simulink library "ddm"  (R2021b)
settings: Solver=VariableStepAuto  StartTime=0.0  StopTime=10.0  RelTol=1e-3
undefined symbols (not defined in the file): ADDM_FrTMTqDev_X_Nm, ADDM_RrTMTqDev_X_Nm, ENUM_ADASACCSTA_ERROR, ENUM_ADASACCSTA_OFF, ENUM_ADASACCSTA_STANDBY, ENUM_ALLOWMOV_ALLOWREADY, ENUM_APS, ENUM_BRKSTA_ERROR, ENUM_BRKSTA_OFF, ENUM_BRKSTA_ON, ENUM_BRKSW_INVALID, ENUM_BRKSW_OFF, ENUM_BRKSW_ON, ENUM_CHGPREACTERRSTA_OBCPRE, ENUM_DCDCFAULTSTA_ANYFAULTLV1, ENUM_DCDCFAULTSTA_ANYFAULTLV2, ENUM_DRIVETRAIN_AWD, ENUM_DRIVETRAIN_FWD, ENUM_DRIVETRAIN_RWD, ENUM_EDUDRTSTA_NORMAL, ENUM_EPBERROR_FAILED, ENUM_EPBSTA_APPLIED, ENUM_EPBSTA_RELEASED, ENUM_ESCAPSSta_APSUNAVAILABLE, ENUM_GEARACTUALPOSN_INVALID, ENUM_GEARACTUALPOSN_P, ENUM_HVBATTREADYPRE_READY, ENUM_HWRESETSTA_HWRESETING, ENUM_MCUWARN_LV0, ENUM_MCUWARN_LV1, ENUM_MCUWARN_LV2, ENUM_MCUWARN_LV3, ENUM_MCUWARN_NOERROR, ENUM_OBCFAULTSTA_ANYFAULT, ENUM_PAS_R2F2, ENUM_PDFAULT_BATTPDFAIL, ENUM_PDFAULT_DCDCDISABLE, ENUM_PDFAULT_MCUDISABLE, ENUM_PDFAULT_MCUDISCHRG, ENUM_POWERSTA_OFF, ENUM_POWERSTA_ON, ENUM_POWERSTA_READY, ENUM_POWERSTA_STANDBY, ENUM_PRESSINDI_LOW, ENUM_PUFAULT_BATTUPFAIL, ENUM_PUFAULT_DCDCENABLEFAIL, ENUM_PUFAULT_PRECHRGCHKFAIL, ENUM_PUFAULT_SAFETYCHKFAIL, ENUM_PWRSTASW_OFF, ENUM_PWRSTASW_OFFA, ENUM_PWRSTASW_OFFCHVCHRG, ENUM_PWRSTASW_OFFCLVCHRG, ENUM_PWRSTASW_ON, ENUM_PWRSTASW_ONHVCHRG, ENUM_PWRSTASW_READY, ENUM_PWRSTASW_STANDBY, ENUM_RAPSErrWarnSta_NORMAL, ENUM_RAPSErrWarnSta_RAPSERRLV1, ENUM_SHIFTCOMMAND_P, ENUM_SHIFTERERRSTA_PBUTTONFAILURE ... (+471)
libraries: hcu_lib x540, simulink x3
(part 10 of 26)

== system ddm/DDM/DDM/PMM/power up and power down ==
  note: VDDM_EDriveSysErrPowerUp_flg
  note: Power up fail check
  note: Power down fail check
  note: OBC ready for precharge fail check
  note: VDDM_EDriveSysErrPowerUp_flg
  note: VDDM_EDriveSysErrPowerUp_flg
  note: VDDM_EDriveSysErrPowerUp_flg
  task_time_s : Inport
  VPMM_PwrStaSW_enum : Inport  Port=2
  VPMM_PowerSta_enum : Inport  Port=3
  VPMM_PowerUpFault_enum : Inport  Port=4
  VPMM_PowerDownFault_enum : Inport  Port=5
  DTC_clear_request : Inport  Port=6
  VINP_HVBattReady4Pre_enum : Inport  Port=7
  VDDM_RrMCUReady4Pre_flg : Inport  Port=8
  VINP_DCDCReady4Pre_flg : Inport  Port=9
  VINP_HVBContactorSta_flg : Inport  Port=10
  VINP_BMSREADY_flg : Inport  Port=11
  VINP_DCDCEnabled_flg : Inport  Port=12
  VPMM_SafetyChkHLv_flg : Inport  Port=13
  VPMM_SafetyChkMLv_flg : Inport  Port=14
  VPMM_HVChrgPreActionErrSta_enum : Inport  Port=15
  VDDM_RrMCUDCBusVolt_V : Inport  Port=16
  VDDM_ClearZevDTCcmd_flg : Inport  Port=17
  VDDM_FrMCUReady4Pre_flg : Inport  Port=18
  VDDM_RrMCUEnaSta_flg : Inport  Port=19
  VDDM_FrMCUEnaSta_flg : Inport  Port=20
  VDDM_FrMCUDCBusVolt_V : Inport  Port=21
  BMS HV relay closed fail : Subsystem
  BMS HV relay opened fail : Subsystem
  BMS ready fail : Subsystem
  DCDC disable fail : Subsystem
  DCDC enable fail : Subsystem
  DCDC ready for precharge fail : Subsystem
  Fr_MCU active discharge fail : Subsystem
  Fr_MCU disable fail : Subsystem
  Fr_MCU ready for precharge fail : Subsystem
  Ground : Ground
  HVB ready for precharge fail : Subsystem
  High level system safety check fail : Subsystem
  Logical Operator : Logic  Operator=OR  AllPortsSameDT=off  OutDataTypeStr=boolean
  Logical Operator1 : Logic  Operator=OR  Inputs=9  AllPortsSameDT=off  OutDataTypeStr=boolean
      settings: AttributesFormatString=%<Operator>
  Logical Operator2 : Logic  Operator=OR  Inputs=3  AllPortsSameDT=off  OutDataTypeStr=boolean
      settings: AttributesFormatString=%<Operator>
  Mid level system safety check fail : Subsystem
  OBC ready for precharge fail : Subsystem
  Rr_MCU active discharge fail : Subsystem
  Rr_MCU disable fail : Subsystem
  Rr_MCU ready for precharge fail : Subsystem
  VDDM_HVB4PreDTC_raw32 : Outport
  VDDM_MCU4PreDTC_raw32 : Outport  Port=2
  VDDM_DCDC4PreDTC_raw32 : Outport  Port=3
  VDDM_HVRlyCloDTC_raw32 : Outport  Port=4
  VDDM_BMSRdyDTC_raw32 : Outport  Port=5
  VDDM_DCDCEnaDTC_raw32 : Outport  Port=6
  VDDM_HiLvSaChkDTC_raw32 : Outport  Port=7
  VDDM_MidLvSaChkDTC_raw32 : Outport  Port=8
  VDDM_MCUDisDTC_raw32 : Outport  Port=9
  VDDM_DCDCDisDTC_raw32 : Outport  Port=10
  VDDM_HVRlyOpDTC_raw32 : Outport  Port=11
  VDDM_MCUActDTC_raw32 : Outport  Port=12
  VDDM_OBC4PreDTC_raw32 : Outport  Port=13
  VDDM_HVRlyOpFail_flg : Outport  Port=14
  VDDM_MCUActDisFail_flg : Outport  Port=15
  VDDM_HVB4PreCFS_flg : Outport  Port=16
  VDDM_RrMCU4PreCFS_flg : Outport  Port=17
  VDDM_DCDC4PreCFS_flg : Outport  Port=18
  VDDM_HVRlyCloCFS_flg : Outport  Port=19
  VDDM_BMSRdyCFS_flg : Outport  Port=20
  VDDM_DCDCEnaCFS_flg : Outport  Port=21
  VDDM_HiLvSaChkCFS_flg : Outport  Port=22
  VDDM_MidLvSaChkCFS_flg : Outport  Port=23
  VDDM_RrMCUDisCFS_flg : Outport  Port=24
  VDDM_DCDCDisCFS_flg : Outport  Port=25
  VDDM_HVRlyOpCFS_flg : Outport  Port=26
  VDDM_RrMCUActCFS_flg : Outport  Port=27
  VDDM_OBC4PreCFS_flg : Outport  Port=28
  VDDM_FrMCU4PreDTC_raw32 : Outport  Port=29
  VDDM_FrMCUDisDTC_ra32 : Outport  Port=30
  VDDM_FrMCUActDTC_raw32 : Outport  Port=31
  VDDM_FrMCU4PreCFS_flg : Outport  Port=32
  VDDM_FrMCUDisCFS_flg : Outport  Port=33
  VDDM_FrMCUActCFS_flg : Outport  Port=34
  VDDM_EDriveSysErrPowerUp_flg : Outport  Port=35
  VDDM_EDriveSysErrPowerDown_flg : Outport  Port=36
  VDDM_SystemPowerUpErr_flg : Outport  Port=37
  VDDM_SystemPowerDownErr_flg : Outport  Port=38
  wires:
  BMS HV relay closed fail/1(VDDM_HVRlyCloDTC_raw32) -> VDDM_HVRlyCloDTC_raw32/1
  DCDC ready for precharge fail/1(VDDM_DCDC4PreDTC_raw32) -> VDDM_DCDC4PreDTC_raw32/1
  Rr_MCU ready for precharge fail/1(VDDM_MCU4PreDTC_raw32) -> VDDM_MCU4PreDTC_raw32/1
  HVB ready for precharge fail/1(VDDM_HVB4PreDTC_raw32) -> VDDM_HVB4PreDTC_raw32/1
  BMS HV relay opened fail/2(VDDM_HVRlyOpFail_flg) -> VDDM_HVRlyOpFail_flg/1
  [VINP_HVBContactorSta_flg] -> BMS HV relay closed fail/4(VINP_HVBContactorSta_flg)
  VINP_HVBContactorSta_flg/1 -> [VINP_HVBContactorSta_flg]
  [VPMM_PowerDownFault_enum] -> Rr_MCU active discharge fail/4(VPMM_PowerDownFault_enum)
  [VPMM_PowerDownFault_enum] -> BMS HV relay opened fail/4(VPMM_PowerDownFault_enum)
  [VPMM_PowerDownFault_enum] -> DCDC disable fail/4(VPMM_PowerDownFault_enum)
  [VINP_DCDCEnabled_flg] -> DCDC enable fail/4(VINP_DCDCEnabled_flg)
  VINP_DCDCEnabled_flg/1 -> [VINP_DCDCEnabled_flg]
  [VPMM_PowerDownFault_enum] -> Rr_MCU disable fail/4(VPMM_PowerDownFault_enum)
  VPMM_PowerDownFault_enum/1 -> [VPMM_PowerDownFault_enum]
  [VPMM_PowerUpFault_enum] -> Mid level system safety check fail/5(VPMM_PowerUpFault_enum)
  VPMM_SafetyChkMLv_flg/1 -> Mid level system safety check fail/4(VDDM_MidLvSaChkChk_flg)
  High level system safety check fail/1(VDDM_HiLvSaChkDTC_raw32) -> VDDM_HiLvSaChkDTC_raw32/1
  VPMM_SafetyChkHLv_flg/1 -> High level system safety check fail/4(VPMM_SafetyChkHLv_flg)
  [VPMM_PowerSta_enum] -> High level system safety check fail/3(VPMM_PwrStaSW_enum)
  [DTC_clear_request] -> High level system safety check fail/6(DTC_clear_request)
  [VPMM_PowerUpFault_enum] -> High level system safety check fail/5(VPMM_PowerUpFault_enum)
  [VPMM_PwrStaSW_enum] -> High level system safety check fail/2(VPMM_PowerSta_enum)
  [task_time_s] -> High level system safety check fail/1(task_time_s)
  DCDC enable fail/1(VDDM_DCDCEnaDTC_raw32) -> VDDM_DCDCEnaDTC_raw32/1
  [VPMM_PowerSta_enum] -> DCDC enable fail/3(VPMM_PwrStaSW_enum)
  [VPMM_PwrStaSW_enum] -> DCDC enable fail/2(VPMM_PowerSta_enum)
  [VDDM_ClearZevDTCcmd_flg] -> DCDC enable fail/6(DTC_clear_request)
  [VPMM_PowerUpFault_enum] -> DCDC enable fail/5(VPMM_PowerUpFault_enum)
  [task_time_s] -> DCDC enable fail/1(task_time_s)
  BMS ready fail/1(VDDM_BMSRdyDTC_raw32) -> VDDM_BMSRdyDTC_raw32/1
  VINP_BMSREADY_flg/1 -> BMS ready fail/4(VINP_BMSREADY_flg)
  [VPMM_PowerSta_enum] -> BMS ready fail/3(VPMM_PwrStaSW_enum)
  [VPMM_PwrStaSW_enum] -> BMS ready fail/2(VPMM_PowerSta_enum)
  [VDDM_ClearZevDTCcmd_flg] -> BMS ready fail/6(DTC_clear_request)
  [VPMM_PowerUpFault_enum] -> BMS ready fail/5(VPMM_PowerUpFault_enum)
  [task_time_s] -> BMS ready fail/1(task_time_s)
  [VPMM_PowerUpFault_enum] -> BMS HV relay closed fail/5(VPMM_PowerUpFault_enum)
  [VPMM_PowerUpFault_enum] -> DCDC ready for precharge fail/5(VPMM_PowerUpFault_enum)
  [VPMM_PowerUpFault_enum] -> Rr_MCU ready for precharge fail/4(VPMM_PowerUpFault_enum)
  [VDDM_ClearZevDTCcmd_flg] -> Rr_MCU ready for precharge fail/5(DTC_clear_request)
  [VPMM_PowerUpFault_enum] -> HVB ready for precharge fail/5(VPMM_PowerUpFault_enum)
  VPMM_HVChrgPreActionErrSta_enum/1 -> OBC ready for precharge fail/4(VPMM_HVChrgPreActionErrSta_enum)
  VINP_DCDCReady4Pre_flg/1 -> DCDC ready for precharge fail/4(VINP_DCDCReady4Pre_flg)
  VINP_HVBattReady4Pre_enum/1 -> HVB ready for precharge fail/4(VINP_HVBattReady4Pre_enum)
  Rr_MCU active discharge fail/1(VDDM_MCUActDTC_raw32) -> VDDM_MCUActDTC_raw32/1
  Rr_MCU disable fail/1(VDDM_MCUDisDTC_raw32) -> VDDM_MCUDisDTC_raw32/1
  Mid level system safety check fail/1(VDDM_MidLvSaChkDTC_raw32) -> VDDM_MidLvSaChkDTC_raw32/1
  BMS HV relay opened fail/1(VDDM_HVRlyOpDTC_raw32) -> VDDM_HVRlyOpDTC_raw32/1
  OBC ready for precharge fail/1(VDDM_OBC4PreDTC_raw32) -> VDDM_OBC4PreDTC_raw32/1
  DCDC disable fail/1(VDDM_DCDCDisDTC_raw32) -> VDDM_DCDCDisDTC_raw32/1
  [VDDM_ClearZevDTCcmd_flg] -> OBC ready for precharge fail/5(DTC_clear_request)
  [task_time_s] -> OBC ready for precharge fail/1(task_time_s)
  [task_time_s] -> Rr_MCU active discharge fail/1(task_time_s)
  [VPMM_PwrStaSW_enum] -> Rr_MCU active discharge fail/3(VPMM_PwrStaSW_enum)
  [VDDM_ClearZevDTCcmd_flg] -> Rr_MCU active discharge fail/5(DTC_clear_request)
  [VPMM_PowerSta_enum] -> Rr_MCU active discharge fail/2(VPMM_PowerSta_enum)
  [VPMM_PowerSta_enum] -> BMS HV relay opened fail/2(VPMM_PowerSta_enum)
  [VDDM_ClearZevDTCcmd_flg] -> BMS HV relay opened fail/5(DTC_clear_request)
  [VPMM_PwrStaSW_enum] -> BMS HV relay opened fail/3(VPMM_PwrStaSW_enum)
  [task_time_s] -> BMS HV relay opened fail/1(task_time_s)
  [task_time_s] -> DCDC disable fail/1(task_time_s)
  [VDDM_ClearZevDTCcmd_flg] -> DCDC disable fail/5(DTC_clear_request)
  [VPMM_PowerSta_enum] -> Rr_MCU disable fail/2(VPMM_PowerSta_enum)
  [VDDM_ClearZevDTCcmd_flg] -> Rr_MCU disable fail/5(DTC_clear_request)
  [VPMM_PwrStaSW_enum] -> Rr_MCU disable fail/3(VPMM_PwrStaSW_enum)
  [task_time_s] -> Rr_MCU disable fail/1(task_time_s)
  [task_time_s] -> Mid level system safety check fail/1(task_time_s)
  [VPMM_PwrStaSW_enum] -> Mid level system safety check fail/2(VPMM_PowerSta_enum)
  [DTC_clear_request] -> Mid level system safety check fail/6(DTC_clear_request)
  [VPMM_PowerSta_enum] -> Mid level system safety check fail/3(VPMM_PwrStaSW_enum)
  DTC_clear_request/1 -> [DTC_clear_request]
  VPMM_PowerSta_enum/1 -> [VPMM_PowerSta_enum]
  task_time_s/1 -> [task_time_s]
  VPMM_PwrStaSW_enum/1 -> [VPMM_PwrStaSW_enum]
  VPMM_PowerUpFault_enum/1 -> [VPMM_PowerUpFault_enum]
  [task_time_s] -> Rr_MCU ready for precharge fail/1(task_time_s)
  [VPMM_PwrStaSW_enum] -> HVB ready for precharge fail/2(VPMM_PowerSta_enum)
  [VPMM_PwrStaSW_enum] -> BMS HV relay closed fail/2(VPMM_PowerSta_enum)
  [VPMM_PowerSta_enum] -> BMS HV relay closed fail/3(VPMM_PwrStaSW_enum)
  [task_time_s] -> BMS HV relay closed fail/1(task_time_s)
  [VPMM_PowerSta_enum] -> Rr_MCU ready for precharge fail/3(VPMM_PwrStaSW_enum)
  [VPMM_PwrStaSW_enum] -> DCDC ready for precharge fail/2(VPMM_PowerSta_enum)
  [task_time_s] -> DCDC ready for precharge fail/1(task_time_s)
  [VDDM_ClearZevDTCcmd_flg] -> DCDC ready for precharge fail/6(VINP_ReqClrDTC_flg)
  [task_time_s] -> HVB ready for precharge fail/1(task_time_s)
  [VDDM_ClearZevDTCcmd_flg] -> HVB ready for precharge fail/6(DTC_clear_request)
  [VPMM_PowerSta_enum] -> HVB ready for precharge fail/3(VPMM_PwrStaSW_enum)
  [VPMM_PowerSta_enum] -> DCDC ready for precharge fail/3(VPMM_PwrStaSW_enum)
  [VPMM_PwrStaSW_enum] -> Rr_MCU ready for precharge fail/2(VPMM_PowerSta_enum)
  [VDDM_ClearZevDTCcmd_flg] -> BMS HV relay closed fail/6(DTC_clear_request)
  [VDDM_RrMCUDCBusVolt_V] -> Rr_MCU active discharge fail/6(VDDM_RrMCUDCBusVolt_V)
  HVB ready for precharge fail/2(VDDM_HVB4PreCFS_flg) -> [VDDM_HVB4PreCFS_flg]
  Rr_MCU ready for precharge fail/2(VDDM_RrMCU4PreCFS_flg) -> [VDDM_RrMCU4PreCFS_flg]
  DCDC ready for precharge fail/2(VDDM_DCDC4PreCFS_flg) -> [VDDM_DCDC4PreCFS_flg]
  BMS HV relay closed fail/2(VDDM_HVRlyCloCFS_flg) -> [VDDM_HVRlyCloCFS_flg]
  BMS ready fail/2(VDDM_BMSRdyCFS_flg) -> [VDDM_BMSRdyCFS_flg]
  DCDC enable fail/2(VDDM_DCDCEnaCFS_flg) -> [VDDM_DCDCEnaCFS_flg]
  High level system safety check fail/2(VDDM_HiLvSaChkCFS_flg) -> [VDDM_HiLvSaChkCFS_flg]
  Mid level system safety check fail/2(VDDM_MidLvSaChkCFS_flg) -> [VDDM_MidLvSaChkCFS_flg]
  Rr_MCU disable fail/2(VDDM_RrMCUDisCFS_flg) -> [VDDM_RrMCUDisCFS_flg]
  DCDC disable fail/2(VDDM_DCDCDisCFS_flg) -> [VDDM_DCDCDisCFS_flg]
  BMS HV relay opened fail/3(VDDM_HVRlyOpCFS_flg) -> [VDDM_HVRlyOpCFS_flg]
  Rr_MCU active discharge fail/3(VDDM_RrMCUActCFS_flg) -> [VDDM_RrMCUActCFS_flg]
  OBC ready for precharge fail/2(VDDM_OBC4PreCFS_flg) -> [VDDM_OBC4PreCFS_flg]
  [VDDM_HVB4PreCFS_flg] -> VDDM_HVB4PreCFS_flg/1
  [VDDM_RrMCU4PreCFS_flg] -> VDDM_RrMCU4PreCFS_flg/1
  [VDDM_DCDC4PreCFS_flg] -> VDDM_DCDC4PreCFS_flg/1
  [VDDM_HVRlyCloCFS_flg] -> VDDM_HVRlyCloCFS_flg/1
  [VDDM_BMSRdyCFS_flg] -> VDDM_BMSRdyCFS_flg/1
  [VDDM_DCDCEnaCFS_flg] -> VDDM_DCDCEnaCFS_flg/1
  [VDDM_HiLvSaChkCFS_flg] -> VDDM_HiLvSaChkCFS_flg/1
  [VDDM_MidLvSaChkCFS_flg] -> VDDM_MidLvSaChkCFS_flg/1
  [VDDM_RrMCUDisCFS_flg] -> VDDM_RrMCUDisCFS_flg/1
  [VDDM_DCDCDisCFS_flg] -> VDDM_DCDCDisCFS_flg/1
  [VDDM_HVRlyOpCFS_flg] -> VDDM_HVRlyOpCFS_flg/1
  [VDDM_RrMCUActCFS_flg] -> VDDM_RrMCUActCFS_flg/1
  [VDDM_OBC4PreCFS_flg] -> VDDM_OBC4PreCFS_flg/1
  VDDM_RrMCUDCBusVolt_V/1 -> [VDDM_RrMCUDCBusVolt_V]
  VDDM_ClearZevDTCcmd_flg/1 -> [VDDM_ClearZevDTCcmd_flg]
  [VDDM_FrMCUReady4Pre_flg] -> Fr_MCU ready for precharge fail/6(VDDM_FrMCUReady4Pre_flg)
  [DTC_clear_request] -> Fr_MCU ready for precharge fail/5(DTC_clear_request)
  [VPMM_PowerSta_enum] -> Fr_MCU ready for precharge fail/3(VPMM_PwrStaSW_enum)
  [task_time_s] -> Fr_MCU ready for precharge fail/1(task_time_s)
  Fr_MCU ready for precharge fail/2(VDDM_FrMCU4PreCFS_flg) -> [VDDM_FrMCU4PreCFS_flg]
  [VPMM_PowerUpFault_enum] -> Fr_MCU ready for precharge fail/4(VPMM_PowerUpFault_enum)
  [VPMM_PwrStaSW_enum] -> Fr_MCU ready for precharge fail/2(VPMM_PowerSta_enum)
  Fr_MCU ready for precharge fail/1(VDDM_FrMCU4PreDTC_raw32) -> VDDM_FrMCU4PreDTC_raw32/1
  Ground/1 -> [VPMM_PowerUpState_enum]
  [VDDM_RrMCUEnaSta_flg] -> Rr_MCU disable fail/6(VDDM_RrMCUEnaSta_flg)
  [VPMM_PowerSta_enum] -> DCDC disable fail/2(VPMM_PowerSta_enum)
  [VPMM_PwrStaSW_enum] -> DCDC disable fail/3(VPMM_PwrStaSW_enum)
  Rr_MCU active discharge fail/2(VDDM_RrMCUActDisFail_flg) -> [VDDM_RrMCUActDisFail_flg]
  [VPMM_PowerSta_enum] -> Fr_MCU disable fail/3(VPMM_PwrStaSW_enum)
  [task_time_s] -> Fr_MCU disable fail/1(task_time_s)
  [VDDM_FrMCUEnaSta_flg] -> Fr_MCU disable fail/6(VDDM_FrMCUEnaSta_flg)
  Fr_MCU disable fail/1(VDDM_FrMCUDisDTC_raw32) -> VDDM_FrMCUDisDTC_ra32/1
  [DTC_clear_request] -> Fr_MCU disable fail/5(DTC_clear_request)
  Fr_MCU disable fail/2(VDDM_FrMCUDisCFS_flg) -> [VDDM_FrMCUDisCFS_flg]
  [VPMM_PowerDownFault_enum] -> Fr_MCU disable fail/4(VPMM_PowerDownFault_enum)
  [VPMM_PwrStaSW_enum] -> Fr_MCU disable fail/2(VPMM_PowerSta_enum)
  [VPMM_PwrStaSW_enum] -> Fr_MCU active discharge fail/3(VPMM_PwrStaSW_enum)
  Fr_MCU active discharge fail/2(VDDM_FrMCUActDisFail_flg) -> [VDDM_FrMCUActDisFail_flg]
  [VPMM_PowerSta_enum] -> Fr_MCU active discharge fail/2(VPMM_PowerSta_enum)
  [task_time_s] -> Fr_MCU active discharge fail/1(task_time_s)
  [DTC_clear_request] -> Fr_MCU active discharge fail/5(DTC_clear_request)
  Fr_MCU active discharge fail/3(VDDM_FrMCUActCFS_flg) -> [VDDM_FrMCUActCFS_flg]
  Fr_MCU active discharge fail/1(VDDM_FrMCUActDTC_raw32) -> VDDM_FrMCUActDTC_raw32/1
  [VDDM_FrMCUDCBusVolt_V] -> Fr_MCU active discharge fail/6(VDDM_FrMCUDCBusVolt_V)
  [VPMM_PowerDownFault_enum] -> Fr_MCU active discharge fail/4(VPMM_PowerDownFault_enum)
  [VDDM_RrMCUActDisFail_flg] -> Logical Operator/2
  [VDDM_FrMCUActDisFail_flg] -> Logical Operator/1
  Logical Operator/1 -> VDDM_MCUActDisFail_flg/1  "VDDM_MCUActDisFail_flg"
  [VPMM_PowerSta_enum] -> OBC ready for precharge fail/2(VPMM_PowerSta_enum)
  [VPMM_PwrStaSW_enum] -> OBC ready for precharge fail/3(VPMM_PwrStaSW_enum)
  [VDDM_FrMCUDisCFS_flg] -> VDDM_FrMCUDisCFS_flg/1
  [VDDM_FrMCU4PreCFS_flg] -> VDDM_FrMCU4PreCFS_flg/1
  [VDDM_FrMCUActCFS_flg] -> VDDM_FrMCUActCFS_flg/1
  Logical Operator2/1 -> [VDDM_EDriveSysErrPowerDown_flg], [VDDM_SystemPowerDownErr_flg]  "VDDM_EDriveSysErrPowerDown_flg"
  [VDDM_FrMCU4PreCFS_flg] -> Logical Operator1/3
  [VDDM_FrMCUActCFS_flg] -> Logical Operator2/2
  [VDDM_HVRlyOpCFS_flg] -> Logical Operator2/1
  [VDDM_MidLvSaChkCFS_flg] -> Logical Operator1/9
  [VDDM_DCDC4PreCFS_flg] -> Logical Operator1/4
  [VDDM_HVRlyCloCFS_flg] -> Logical Operator1/5
  Logical Operator1/1 -> [VDDM_EDriveSysErrPowerUp_flg], [VDDM_SystemPowerUpErr_flg]  "VDDM_EDriveSysErrPowerUp_flg"
  [VDDM_HiLvSaChkCFS_flg] -> Logical Operator1/8
  [VDDM_HVB4PreCFS_flg] -> Logical Operator1/1
  [VDDM_BMSRdyCFS_flg] -> Logical Operator1/6
  [VDDM_DCDCEnaCFS_flg] -> Logical Operator1/7
  [VDDM_RrMCUActCFS_flg] -> Logical Operator2/3
  [VDDM_RrMCU4PreCFS_flg] -> Logical Operator1/2
  [VDDM_EDriveSysErrPowerUp_flg] -> VDDM_EDriveSysErrPowerUp_flg/1
  [VDDM_EDriveSysErrPowerDown_flg] -> VDDM_EDriveSysErrPowerDown_flg/1
  [VDDM_RrMCUReady4Pre_flg] -> Rr_MCU ready for precharge fail/6(VDDM_RrMCUReady4Pre_flg)
  VDDM_RrMCUReady4Pre_flg/1 -> [VDDM_RrMCUReady4Pre_flg]
  VDDM_FrMCUReady4Pre_flg/1 -> [VDDM_FrMCUReady4Pre_flg]
  VDDM_RrMCUEnaSta_flg/1 -> [VDDM_RrMCUEnaSta_flg]
  VDDM_FrMCUEnaSta_flg/1 -> [VDDM_FrMCUEnaSta_flg]
  VDDM_FrMCUDCBusVolt_V/1 -> [VDDM_FrMCUDCBusVolt_V]
  [VDDM_SystemPowerDownErr_flg] -> VDDM_SystemPowerDownErr_flg/1
  [VDDM_SystemPowerUpErr_flg] -> VDDM_SystemPowerUpErr_flg/1

== system ddm/DDM/DDM/Subsystem/Subsystem ==
  VPMM_SysPwrSta_enum : Inport
  VINP_CANBusError_flg : Inport  Port=2
  Constant17 : Constant  Value=ENUM_PWRSTASW_READY
  Constant3 : Constant  Value=ENUM_PWRSTASW_ON
  Equal2 : RelationalOperator  Operator===  OutDataTypeStr=boolean  RndMeth=Simplest
  Equal6 : RelationalOperator  Operator===  OutDataTypeStr=boolean  RndMeth=Simplest
  Logical Operator1 : Logic  AllPortsSameDT=off  OutDataTypeStr=boolean
  Logical Operator13 : Logic  Operator=OR  AllPortsSameDT=off  OutDataTypeStr=boolean
  Logical Operator2 : Logic  AllPortsSameDT=off  OutDataTypeStr=boolean
  NOT : Logic  Operator=NOT  AllPortsSameDT=off  OutDataTypeStr=boolean
  VDDM_CANBusErrorPass_flg : Outport
  VDDM_CANBusErrorCFS_flg : Outport  Port=2
  wires:
  Equal6/1 -> Logical Operator13/1
  [VPMM_SysPwrSta_enum] -> Equal6/1
  Equal2/1 -> Logical Operator13/2
  [VPMM_SysPwrSta_enum] -> Equal2/1
  Constant3/1 -> Equal6/2
  Constant17/1 -> Equal2/2
  VPMM_SysPwrSta_enum/1 -> [VPMM_SysPwrSta_enum]
  VINP_CANBusError_flg/1 -> [VINP_CANBusError_flg]
  Logical Operator13/1 -> Logical Operator2/1, Logical Operator1/1
  [VINP_CANBusError_flg] -> NOT/1, Logical Operator1/2
  Logical Operator1/1 -> VDDM_CANBusErrorCFS_flg/1
  NOT/1 -> Logical Operator2/2
  Logical Operator2/1 -> VDDM_CANBusErrorPass_flg/1

== system ddm/DDM/DDM/Subsystem/Subsystem1 ==
  VPMM_SysPwrSta_enum : Inport
  VINP_CANBusError_flg : Inport  Port=2
  Constant17 : Constant  Value=ENUM_PWRSTASW_READY
  Constant3 : Constant  Value=ENUM_PWRSTASW_ON
  Equal2 : RelationalOperator  Operator===  OutDataTypeStr=boolean  RndMeth=Simplest
  Equal6 : RelationalOperator  Operator===  OutDataTypeStr=boolean  RndMeth=Simplest
  Logical Operator1 : Logic  AllPortsSameDT=off  OutDataTypeStr=boolean
  Logical Operator13 : Logic  Operator=OR  AllPortsSameDT=off  OutDataTypeStr=boolean
  Logical Operator2 : Logic  AllPortsSameDT=off  OutDataTypeStr=boolean
  NOT : Logic  Operator=NOT  AllPortsSameDT=off  OutDataTypeStr=boolean
  VDDM_CANBusErrorPass_flg : Outport
  VDDM_CANBusErrorCFS_flg : Outport  Port=2
  wires:
  Logical Operator2/1 -> VDDM_CANBusErrorPass_flg/1
  NOT/1 -> Logical Operator2/2
  Logical Operator1/1 -> VDDM_CANBusErrorCFS_flg/1
  [VINP_CANBusError_flg] -> Logical Operator1/2, NOT/1
  Logical Operator13/1 -> Logical Operator1/1, Logical Operator2/1
  VINP_CANBusError_flg/1 -> [VINP_CANBusError_flg]
  VPMM_SysPwrSta_enum/1 -> [VPMM_SysPwrSta_enum]
  Constant17/1 -> Equal2/2
  Constant3/1 -> Equal6/2
  [VPMM_SysPwrSta_enum] -> Equal2/1
  Equal2/1 -> Logical Operator13/2
  [VPMM_SysPwrSta_enum] -> Equal6/1
  Equal6/1 -> Logical Operator13/1

== system ddm/DDM/DDM/Subsystem/Subsystem2 ==
  VPMM_SysPwrSta_enum : Inport
  VINP_CANBusError_flg : Inport  Port=2
  Constant17 : Constant  Value=ENUM_PWRSTASW_READY
  Constant3 : Constant  Value=ENUM_PWRSTASW_ON
  Equal2 : RelationalOperator  Operator===  OutDataTypeStr=boolean  RndMeth=Simplest
  Equal6 : RelationalOperator  Operator===  OutDataTypeStr=boolean  RndMeth=Simplest
  Logical Operator1 : Logic  AllPortsSameDT=off  OutDataTypeStr=boolean
  Logical Operator13 : Logic  Operator=OR  AllPortsSameDT=off  OutDataTypeStr=boolean
  Logical Operator2 : Logic  AllPortsSameDT=off  OutDataTypeStr=boolean
  NOT : Logic  Operator=NOT  AllPortsSameDT=off  OutDataTypeStr=boolean
  VDDM_CANBusErrorPass_flg : Outport
  VDDM_CANBusErrorCFS_flg : Outport  Port=2
  wires:
  Logical Operator2/1 -> VDDM_CANBusErrorPass_flg/1
  NOT/1 -> Logical Operator2/2
  Logical Operator1/1 -> VDDM_CANBusErrorCFS_flg/1
  [VINP_CANBusError_flg] -> Logical Operator1/2, NOT/1
  Logical Operator13/1 -> Logical Operator1/1, Logical Operator2/1
  VINP_CANBusError_flg/1 -> [VINP_CANBusError_flg]
  VPMM_SysPwrSta_enum/1 -> [VPMM_SysPwrSta_enum]
  Constant17/1 -> Equal2/2
  Constant3/1 -> Equal6/2
  [VPMM_SysPwrSta_enum] -> Equal2/1
  Equal2/1 -> Logical Operator13/2
  [VPMM_SysPwrSta_enum] -> Equal6/1
  Equal6/1 -> Logical Operator13/1

== system ddm/DDM/DDM/Subsystem/Subsystem3 ==
  VPMM_SysPwrSta_enum : Inport
  VINP_CANBusError_flg : Inport  Port=2
  Constant17 : Constant  Value=ENUM_PWRSTASW_READY
  Constant3 : Constant  Value=ENUM_PWRSTASW_ON
  Equal2 : RelationalOperator  Operator===  OutDataTypeStr=boolean  RndMeth=Simplest
  Equal6 : RelationalOperator  Operator===  OutDataTypeStr=boolean  RndMeth=Simplest
  Logical Operator1 : Logic  AllPortsSameDT=off  OutDataTypeStr=boolean
  Logical Operator13 : Logic  Operator=OR  AllPortsSameDT=off  OutDataTypeStr=boolean
  Logical Operator2 : Logic  AllPortsSameDT=off  OutDataTypeStr=boolean
  NOT : Logic  Operator=NOT  AllPortsSameDT=off  OutDataTypeStr=boolean
  VDDM_CANBusErrorPass_flg : Outport
  VDDM_CANBusErrorCFS_flg : Outport  Port=2
  wires:
  Logical Operator2/1 -> VDDM_CANBusErrorPass_flg/1
  NOT/1 -> Logical Operator2/2
  Logical Operator1/1 -> VDDM_CANBusErrorCFS_flg/1
  [VINP_CANBusError_flg] -> Logical Operator1/2, NOT/1
  Logical Operator13/1 -> Logical Operator1/1, Logical Operator2/1
  VINP_CANBusError_flg/1 -> [VINP_CANBusError_flg]
  VPMM_SysPwrSta_enum/1 -> [VPMM_SysPwrSta_enum]
  Constant17/1 -> Equal2/2
  Constant3/1 -> Equal6/2
  [VPMM_SysPwrSta_enum] -> Equal2/1
  Equal2/1 -> Logical Operator13/2
  [VPMM_SysPwrSta_enum] -> Equal6/1
  Equal6/1 -> Logical Operator13/1

== system ddm/DDM/DDM/Subsystem/Subsystem4 ==
  VPMM_SysPwrSta_enum : Inport
  VINP_CANBusError_flg : Inport  Port=2
  Constant17 : Constant  Value=ENUM_PWRSTASW_READY
  Constant3 : Constant  Value=ENUM_PWRSTASW_ON
  Equal2 : RelationalOperator  Operator===  OutDataTypeStr=boolean  RndMeth=Simplest
  Equal6 : RelationalOperator  Operator===  OutDataTypeStr=boolean  RndMeth=Simplest
  Logical Operator1 : Logic  AllPortsSameDT=off  OutDataTypeStr=boolean
  Logical Operator13 : Logic  Operator=OR  AllPortsSameDT=off  OutDataTypeStr=boolean
  Logical Operator2 : Logic  AllPortsSameDT=off  OutDataTypeStr=boolean
  NOT : Logic  Operator=NOT  AllPortsSameDT=off  OutDataTypeStr=boolean
  VDDM_CANBusErrorPass_flg : Outport
  VDDM_CANBusErrorCFS_flg : Outport  Port=2
  wires:
  Logical Operator2/1 -> VDDM_CANBusErrorPass_flg/1
  NOT/1 -> Logical Operator2/2
  Logical Operator1/1 -> VDDM_CANBusErrorCFS_flg/1
  [VINP_CANBusError_flg] -> Logical Operator1/2, NOT/1
  Logical Operator13/1 -> Logical Operator1/1, Logical Operator2/1
  VINP_CANBusError_flg/1 -> [VINP_CANBusError_flg]
  VPMM_SysPwrSta_enum/1 -> [VPMM_SysPwrSta_enum]
  Constant17/1 -> Equal2/2
  Constant3/1 -> Equal6/2
  [VPMM_SysPwrSta_enum] -> Equal2/1
  Equal2/1 -> Logical Operator13/2
  [VPMM_SysPwrSta_enum] -> Equal6/1
  Equal6/1 -> Logical Operator13/1

== system ddm/DDM/DDM/Subsystem/Subsystem5 ==
  VPMM_SysPwrSta_enum : Inport
  VINP_CANBusError_flg : Inport  Port=2
  Constant17 : Constant  Value=ENUM_PWRSTASW_READY
  Constant3 : Constant  Value=ENUM_PWRSTASW_ON
  Equal2 : RelationalOperator  Operator===  OutDataTypeStr=boolean  RndMeth=Simplest
  Equal6 : RelationalOperator  Operator===  OutDataTypeStr=boolean  RndMeth=Simplest
  Logical Operator1 : Logic  AllPortsSameDT=off  OutDataTypeStr=boolean
  Logical Operator13 : Logic  Operator=OR  AllPortsSameDT=off  OutDataTypeStr=boolean
  Logical Operator2 : Logic  AllPortsSameDT=off  OutDataTypeStr=boolean
  NOT : Logic  Operator=NOT  AllPortsSameDT=off  OutDataTypeStr=boolean
  VDDM_CANBusErrorPass_flg : Outport
  VDDM_CANBusErrorCFS_flg : Outport  Port=2
  wires:
  Logical Operator2/1 -> VDDM_CANBusErrorPass_flg/1
  NOT/1 -> Logical Operator2/2
  Logical Operator1/1 -> VDDM_CANBusErrorCFS_flg/1
  [VINP_CANBusError_flg] -> Logical Operator1/2, NOT/1
  Logical Operator13/1 -> Logical Operator1/1, Logical Operator2/1
  VINP_CANBusError_flg/1 -> [VINP_CANBusError_flg]
  VPMM_SysPwrSta_enum/1 -> [VPMM_SysPwrSta_enum]
  Constant17/1 -> Equal2/2
  Constant3/1 -> Equal6/2
  [VPMM_SysPwrSta_enum] -> Equal2/1
  Equal2/1 -> Logical Operator13/2
  [VPMM_SysPwrSta_enum] -> Equal6/1
  Equal6/1 -> Logical Operator13/1

== system ddm/DDM/DDM/TPM/LFBatwarn ==
  note: Test Detection Criteria
  note: Test Pass Criteria
  note: Release Condition After Decision
  note: Diagnostics and Fault Handling
  task_time_s : Inport
  VPMM_PowerSta_enum : Inport  Port=2
  DTC_clear_request : Inport  Port=3
  VTPM_LFBatwarn_flg : Inport  Port=4
  Constant : Constant  Value=KDDM_LFBatwarnDTC_cnt
  Constant1 : Constant  Value=KDDM_LFBatwarnDTC_cnt
  Constant10 : Constant  Value=ENUM_POWERSTA_OFF
  Constant11 : Constant  Value=KDDM_LFBatwarnPassSW_flg
  Constant12 : Constant  Value=FALSE
  Constant13 : Constant  Value=KDDM_LFBatwarnCFSSW_flg
  Constant14 : Constant  Value=KDDM_LFBatwarnDFSSW_flg
  Constant15 : Constant  Value=KDDM_LFBatwarnPassTO_s
  Constant2 : Constant  Value=ENUM_POWERSTA_READY
  Constant24 : Constant  Value=TRUE
  Constant25 : Constant  Value=FALSE
  Constant3 : Constant  Value=ENUM_POWERSTA_ON
  Constant4 : Constant  Value=FALSE
  Constant46 : Constant  Value=KDDM_LFBatwarnDetSW_flg
  Constant5 : Constant  Value=ENUM_POWERSTA_READY
  Constant6 : Constant  Value=KDDM_LFBatwarnDetTO_s
  Constant7 : Constant  Value=ENUM_POWERSTA_ON
  Constant8 : Constant  Value=TRUE
  Constant9 : Constant  Value=KDDM_LFBatwarnPassTO_s
  DTC_Couter : hcu_lib/Basic_Blocks/DTC_Couter
  DTC_Info : hcu_lib/Basic_Blocks/DTC_Info
  Data Type Conversion1 : DataTypeConversion  OutDataTypeStr=uint8
  Equal{1..5} (5 alike) : RelationalOperator  Operator===  OutDataTypeStr=boolean  RndMeth=Simplest
  Equal6 : RelationalOperator  OutDataTypeStr=boolean  RndMeth=Simplest
  Logical Operator{1,4..5,7..8} (5 alike) : Logic  Operator=OR  AllPortsSameDT=off  OutDataTypeStr=boolean
  Logical Operator12 : Logic  AllPortsSameDT=off  OutDataTypeStr=boolean
  Logical Operator15 : Logic  AllPortsSameDT=off  OutDataTypeStr=boolean
  Logical Operator18 : Logic  AllPortsSameDT=off  OutDataTypeStr=boolean
  Logical Operator19 : Logic  Inputs=3  AllPortsSameDT=off  OutDataTypeStr=boolean
  Logical Operator2 : Logic  Operator=NOT  AllPortsSameDT=off  OutDataTypeStr=boolean
  Logical Operator3 : Logic  Operator=OR  Inputs=3  AllPortsSameDT=off  OutDataTypeStr=boolean
  Logical Operator6 : Logic  Operator=NOT  AllPortsSameDT=off  OutDataTypeStr=boolean
  Relay : Relay  OnSwitchValue=ONE_INT  OffSwitchValue=ZERO_INT
  SR_Latch1 : Subsystem  mask(SR_Latch){}
      mask help: SR latch function.
  SR_Latch3 : hcu_lib/Basic_Blocks/SR_Latch
  SR_Latch4 : hcu_lib/Basic_Blocks/SR_Latch
  Switch{2..4,6} (4 alike) : Switch  Criteria=u2 ~= 0
  Test Detection Criteria : hcu_lib/Basic_Blocks/Test Detection Criteria
  Timer1 : hcu_lib/Basic_Blocks/Timer
  VDDM_LFBatwarnDTC_raw32 : Outport
  wires:
  task_time_s/1 -> [task_time_s]
  VPMM_PowerSta_enum/1 -> [VPMM_PowerSta_enum]
  Logical Operator8/1 -> Switch2/2
  Constant25/1 -> Switch2/3
  Switch2/1 -> [VDDM_LFBatwarnCFSRls_flg]
  [DTC_clear_request] -> Logical Operator8/2
  Constant24/1 -> Switch2/1
  Constant10/1 -> Equal4/2
  Equal4/1 -> Logical Operator8/1
  [VDDM_LFBatwarnDTC_cnt] -> Relay/1
  [VDDM_LFBatwarnCFS_flg] -> Logical Operator7/1
  Logical Operator3/1 -> Logical Operator15/1
  [VDDM_LFBatwarnDet_flg] -> Logical Operator19/1
  Relay/1 -> SR_Latch3/1
  DTC_Couter/2 -> Data Type Conversion1/1
  Logical Operator15/1 -> DTC_Couter/2
  Constant11/1 -> Logical Operator15/2
  Logical Operator19/1 -> DTC_Couter/1
  Constant46/1 -> Logical Operator19/2
  Data Type Conversion1/1 -> [VDDM_LFBatwarnDTC_cnt]  "VDDM_LFBatwarnDTC_cnt"
  DTC_Couter/1 -> SR_Latch4/1
  [VDDM_LFBatwarnPass_flg] -> Logical Operator3/2
  [VDDM_LFBatwarnCFSRls_flg] -> Logical Operator5/1
  SR_Latch4/1 -> Logical Operator18/1
  Logical Operator12/1 -> [VDDM_LFBatwarnDFS_flg]
  Constant13/1 -> Logical Operator18/2
  SR_Latch3/1 -> Logical Operator12/2
  Constant14/1 -> Logical Operator12/1
  Logical Operator18/1 -> [VDDM_LFBatwarnCFS_flg]
  [VDDM_LFBatwarnCFSRls_flg] -> Logical Operator3/3
  DTC_clear_request/1 -> [DTC_clear_request]
  [VPMM_PowerSta_enum] -> Equal4/1
  [VDDM_LFBatwarnCFS_flg] -> DTC_Info/3
  DTC_Info/1 -> VDDM_LFBatwarnDTC_raw32/1  "VDDM_LFBatwarnDTC_raw32"
  Test Detection Criteria/1 -> [VDDM_LFBatwarnDet_flg]  "VDDM_LFBatwarnDet_flg"
  [VDDM_LFBatwarnDet_flg] -> DTC_Info/1
  [VDDM_LFBatwarnPass_flg] -> DTC_Info/2
  [DTC_clear_request] -> DTC_Info/4
  [VPMM_PowerSta_enum] -> Equal1/1
  Constant4/1 -> Switch3/3
  Constant5/1 -> Equal1/2
  Constant7/1 -> Equal5/2
  Logical Operator1/1 -> Switch3/2
  Equal5/1 -> Logical Operator1/1
  Equal1/1 -> Logical Operator1/2
  [VPMM_PowerSta_enum] -> Equal5/1
  Constant6/1 -> Test Detection Criteria/4
  Constant/1 -> Test Detection Criteria/3
  [task_time_s] -> Test Detection Criteria/2
  [VTPM_LFBatwarn_flg] -> Switch3/1
  [VPMM_PowerSta_enum] -> Equal3/1
  Equal2/1 -> Logical Operator4/2
  Constant8/1 -> Switch4/3
  Constant2/1 -> Equal2/2
  Constant3/1 -> Equal3/2
  [VPMM_PowerSta_enum] -> Equal2/1
  Equal3/1 -> Logical Operator4/1
  Logical Operator4/1 -> Switch4/2
  [VTPM_LFBatwarn_flg] -> Switch4/1
  VTPM_LFBatwarn_flg/1 -> [VTPM_LFBatwarn_flg]
  Switch3/1 -> [VDDM_LFBatwarnChk_flg], Switch6/3
  [DTC_clear_request] -> Switch6/2
  Constant12/1 -> Switch6/1
  Switch6/1 -> Test Detection Criteria/1
  Switch4/1 -> Timer1/2, Logical Operator6/1
  Equal6/1 -> SR_Latch1/1(set)
  Constant9/1 -> Equal6/2
  SR_Latch1/1(latched) -> [VDDM_LFBatwarnPass_flg]
  [VDDM_LFBatwarnChk_flg] -> SR_Latch1/2(reset)
  [task_time_s] -> Timer1/3
  Timer1/1 -> Equal6/1
  Constant15/1 -> Timer1/4
  Logical Operator6/1 -> Timer1/1
  Logical Operator2/1 -> Logical Operator19/3
  [DTC_clear_request] -> Logical Operator3/1, Logical Operator2/1
  Logical Operator5/1 -> SR_Latch4/2
  Constant1/1 -> DTC_Couter/3
  [DTC_clear_request] -> Logical Operator5/2
  [DTC_clear_request] -> Logical Operator7/2
  Logical Operator7/1 -> SR_Latch3/2

== system ddm/DDM/DDM/TPM/LFPressureLow ==
  note: Diagnostics and Fault Handling
  note: Release Condition After Decision
  note: Test Pass Criteria
  note: Test Detection Criteria
  task_time_s : Inport
  VPMM_PowerSta_enum : Inport  Port=2
  DTC_clear_request : Inport  Port=3
  VTPM_LFPressIndi_enum : Inport  Port=4
  Constant : Constant  Value=KDDM_LFPressIndiDTC_cnt
  Constant1 : Constant  Value=KDDM_LFPressIndiDTC_cnt
  Constant10 : Constant  Value=ENUM_POWERSTA_OFF
  Constant11 : Constant  Value=KDDM_LFPressIndiPassSW_flg
  Constant12 : Constant  Value=FALSE
  Constant13 : Constant  Value=KDDM_LFPressIndiCFSSW_flg
  Constant14 : Constant  Value=KDDM_LFPressIndiDFSSW_flg
  Constant15 : Constant  Value=KDDM_LFPressIndiPassTO_s
  Constant16 : Constant  Value=ENUM_PRESSINDI_LOW
  Constant17 : Constant  Value=ENUM_PRESSINDI_LOW
  Constant2 : Constant  Value=ENUM_POWERSTA_READY
  Constant24 : Constant  Value=TRUE
  Constant25 : Constant  Value=FALSE
  Constant3 : Constant  Value=ENUM_POWERSTA_ON
  Constant4 : Constant  Value=FALSE
  Constant46 : Constant  Value=KDDM_LFPressIndiDetSW_flg
  Constant5 : Constant  Value=ENUM_POWERSTA_READY
  Constant6 : Constant  Value=KDDM_LFPressIndiDetTO_s
  Constant7 : Constant  Value=ENUM_POWERSTA_ON
  Constant8 : Constant  Value=TRUE
  Constant9 : Constant  Value=KDDM_LFPressIndiPassTO_s
  DTC_Couter : hcu_lib/Basic_Blocks/DTC_Couter
  DTC_Info : hcu_lib/Basic_Blocks/DTC_Info
  Data Type Conversion1 : DataTypeConversion  OutDataTypeStr=uint8
  Equal{1..5,7..8} (7 alike) : RelationalOperator  Operator===  OutDataTypeStr=boolean  RndMeth=Simplest
  Equal6 : RelationalOperator  OutDataTypeStr=boolean  RndMeth=Simplest
  Logical Operator{1..2,4,7..8} (5 alike) : Logic  Operator=OR  AllPortsSameDT=off  OutDataTypeStr=boolean
  Logical Operator12 : Logic  AllPortsSameDT=off  OutDataTypeStr=boolean
  Logical Operator15 : Logic  AllPortsSameDT=off  OutDataTypeStr=boolean
  Logical Operator18 : Logic  AllPortsSameDT=off  OutDataTypeStr=boolean
  Logical Operator19 : Logic  Inputs=3  AllPortsSameDT=off  OutDataTypeStr=boolean
  Logical Operator3 : Logic  Operator=OR  Inputs=3  AllPortsSameDT=off  OutDataTypeStr=boolean
  Logical Operator5 : Logic  Operator=NOT  AllPortsSameDT=off  OutDataTypeStr=boolean
  Logical Operator6 : Logic  Operator=NOT  AllPortsSameDT=off  OutDataTypeStr=boolean
  Relay : Relay  OnSwitchValue=ONE_INT  OffSwitchValue=ZERO_INT
  SR_Latch1 : Subsystem  mask(SR_Latch){}
      mask help: SR latch function.
  SR_Latch3 : hcu_lib/Basic_Blocks/SR_Latch
  SR_Latch4 : hcu_lib/Basic_Blocks/SR_Latch
  Switch{2..4,6} (4 alike) : Switch  Criteria=u2 ~= 0
  Test Detection Criteria : hcu_lib/Basic_Blocks/Test Detection Criteria
  Timer1 : hcu_lib/Basic_Blocks/Timer
  VDDM_LFPressIndiDTC_raw32 : Outport
  wires:
  Logical Operator6/1 -> Timer1/1
  Constant15/1 -> Timer1/4
  Timer1/1 -> Equal6/1
  [task_time_s] -> Timer1/3
  [VDDM_LFPressIndiChk_flg] -> SR_Latch1/2(reset)
  SR_Latch1/1(latched) -> [VDDM_LFPressIndiPass_flg]
  Constant9/1 -> Equal6/2
  Equal6/1 -> SR_Latch1/1(set)
  Switch4/1 -> Logical Operator6/1, Timer1/2
  Switch6/1 -> Test Detection Criteria/1
  Constant12/1 -> Switch6/1
  [DTC_clear_request] -> Switch6/2
  Switch3/1 -> Switch6/3, [VDDM_LFPressIndiChk_flg]
  VTPM_LFPressIndi_enum/1 -> [VTPM_LFPressIndi_enum]
  Logical Operator4/1 -> Switch4/2
  Equal3/1 -> Logical Operator4/1
  [VPMM_PowerSta_enum] -> Equal2/1
  Constant3/1 -> Equal3/2
  Constant2/1 -> Equal2/2
  Constant8/1 -> Switch4/3
  Equal2/1 -> Logical Operator4/2
  [VPMM_PowerSta_enum] -> Equal3/1
  [task_time_s] -> Test Detection Criteria/2
  Constant/1 -> Test Detection Criteria/3
  Constant6/1 -> Test Detection Criteria/4
  [VPMM_PowerSta_enum] -> Equal5/1
  Equal1/1 -> Logical Operator1/2
  Equal5/1 -> Logical Operator1/1
  Logical Operator1/1 -> Switch3/2
  Constant7/1 -> Equal5/2
  Constant5/1 -> Equal1/2
  Constant4/1 -> Switch3/3
  [VPMM_PowerSta_enum] -> Equal1/1
  [DTC_clear_request] -> DTC_Info/4
  [VDDM_LFPressIndiPass_flg] -> DTC_Info/2
  [VDDM_LFPressIndiDet_flg] -> DTC_Info/1
  Test Detection Criteria/1 -> [VDDM_LFPressIndiDet_flg]  "VDDM_LFPressIndiDet_flg"
  DTC_Info/1 -> VDDM_LFPressIndiDTC_raw32/1  "VDDM_LFPressIndiDTC_raw32"
  [VDDM_LFPressIndiCFS_flg] -> DTC_Info/3
  [VPMM_PowerSta_enum] -> Equal4/1
  DTC_clear_request/1 -> [DTC_clear_request]
  [VDDM_LFPressIndiCFSRls_flg] -> Logical Operator3/3
  Logical Operator18/1 -> [VDDM_LFPressIndiCFS_flg]
  Constant14/1 -> Logical Operator12/1
  SR_Latch3/1 -> Logical Operator12/2
  Constant13/1 -> Logical Operator18/2
  Logical Operator12/1 -> [VDDM_LFPressIndiDFS_flg]
  SR_Latch4/1 -> Logical Operator18/1
  [VDDM_LFPressIndiCFSRls_flg] -> Logical Operator2/1
  [VDDM_LFPressIndiPass_flg] -> Logical Operator3/2
  DTC_Couter/1 -> SR_Latch4/1
  Data Type Conversion1/1 -> [VDDM_LFPressIndiDTC_cnt]  "VDDM_LFPressIndiDTC_cnt"
  Constant46/1 -> Logical Operator19/2
  Logical Operator19/1 -> DTC_Couter/1
  Constant11/1 -> Logical Operator15/2
  Logical Operator15/1 -> DTC_Couter/2
  Constant1/1 -> DTC_Couter/3
  DTC_Couter/2 -> Data Type Conversion1/1
  Relay/1 -> SR_Latch3/1
  [VDDM_LFPressIndiDet_flg] -> Logical Operator19/1
  Logical Operator3/1 -> Logical Operator15/1
  [VDDM_LFPressIndiCFS_flg] -> Logical Operator7/1
  [VDDM_LFPressIndiDTC_cnt] -> Relay/1
  Equal4/1 -> Logical Operator8/1
  Constant10/1 -> Equal4/2
  Constant24/1 -> Switch2/1
  [DTC_clear_request] -> Logical Operator8/2
  Switch2/1 -> [VDDM_LFPressIndiCFSRls_flg]
  Constant25/1 -> Switch2/3
  Logical Operator8/1 -> Switch2/2
  VPMM_PowerSta_enum/1 -> [VPMM_PowerSta_enum]
  task_time_s/1 -> [task_time_s]
  [VTPM_LFPressIndi_enum] -> Equal7/1
  Equal7/1 -> Switch3/1
  Constant16/1 -> Equal7/2
  Equal8/1 -> Switch4/1
  Constant17/1 -> Equal8/2
  [VTPM_LFPressIndi_enum] -> Equal8/1
  Logical Operator5/1 -> Logical Operator19/3
  [DTC_clear_request] -> Logical Operator3/1, Logical Operator5/1
  Logical Operator2/1 -> SR_Latch4/2
  [DTC_clear_request] -> Logical Operator2/2
  Logical Operator7/1 -> SR_Latch3/2
  [DTC_clear_request] -> Logical Operator7/2

== system ddm/DDM/DDM/TPM/LFSensorfail ==
  note: Diagnostics and Fault Handling
  note: Release Condition After Decision
  note: Test Pass Criteria
  note: Test Detection Criteria
  task_time_s : Inport
  VPMM_PowerSta_enum : Inport  Port=2
  DTC_clear_request : Inport  Port=3
  VTPM_LFSensorFail_flg : Inport  Port=4
  Constant : Constant  Value=KDDM_LFSensorFailDTC_cnt
  Constant1 : Constant  Value=KDDM_LFSensorFailDTC_cnt
  Constant10 : Constant  Value=ENUM_POWERSTA_OFF
  Constant11 : Constant  Value=KDDM_LFSensorFailPassSW_flg
  Constant12 : Constant  Value=FALSE
  Constant13 : Constant  Value=KDDM_LFSensorFailCFSSW_flg
  Constant14 : Constant  Value=KDDM_LFSensorFailDFSSW_flg
  Constant15 : Constant  Value=KDDM_LFSensorFailPassTO_s
  Constant2 : Constant  Value=ENUM_POWERSTA_READY
  Constant24 : Constant  Value=TRUE
  Constant25 : Constant  Value=FALSE
  Constant3 : Constant  Value=ENUM_POWERSTA_ON
  Constant4 : Constant  Value=FALSE
  Constant46 : Constant  Value=KDDM_LFSensorFailDetSW_flg
  Constant5 : Constant  Value=ENUM_POWERSTA_READY
  Constant6 : Constant  Value=KDDM_LFSensorFailDetTO_s
  Constant7 : Constant  Value=ENUM_POWERSTA_ON
  Constant8 : Constant  Value=TRUE
  Constant9 : Constant  Value=KDDM_LFSensorFailPassTO_s
  DTC_Couter : hcu_lib/Basic_Blocks/DTC_Couter
  DTC_Info : hcu_lib/Basic_Blocks/DTC_Info
  Data Type Conversion1 : DataTypeConversion  OutDataTypeStr=uint8
  Equal{1..5} (5 alike) : RelationalOperator  Operator===  OutDataTypeStr=boolean  RndMeth=Simplest
  Equal6 : RelationalOperator  OutDataTypeStr=boolean  RndMeth=Simplest
  Logical Operator{1,4..5,7..8} (5 alike) : Logic  Operator=OR  AllPortsSameDT=off  OutDataTypeStr=boolean
  Logical Operator12 : Logic  AllPortsSameDT=off  OutDataTypeStr=boolean
  Logical Operator15 : Logic  AllPortsSameDT=off  OutDataTypeStr=boolean
  Logical Operator18 : Logic  AllPortsSameDT=off  OutDataTypeStr=boolean
  Logical Operator19 : Logic  Inputs=3  AllPortsSameDT=off  OutDataTypeStr=boolean
  Logical Operator2 : Logic  Operator=NOT  AllPortsSameDT=off  OutDataTypeStr=boolean
  Logical Operator3 : Logic  Operator=OR  Inputs=3  AllPortsSameDT=off  OutDataTypeStr=boolean
  Logical Operator6 : Logic  Operator=NOT  AllPortsSameDT=off  OutDataTypeStr=boolean
  Relay : Relay  OnSwitchValue=ONE_INT  OffSwitchValue=ZERO_INT
  SR_Latch1 : Subsystem  mask(SR_Latch){}
      mask help: SR latch function.
  SR_Latch3 : hcu_lib/Basic_Blocks/SR_Latch
  SR_Latch4 : hcu_lib/Basic_Blocks/SR_Latch
  Switch{2..4,6} (4 alike) : Switch  Criteria=u2 ~= 0
  Test Detection Criteria : hcu_lib/Basic_Blocks/Test Detection Criteria
  Timer1 : hcu_lib/Basic_Blocks/Timer
  VDDM_LFSensorFailDTC_raw32 : Outport
  wires:
  Logical Operator6/1 -> Timer1/1
  Constant15/1 -> Timer1/4
  Timer1/1 -> Equal6/1
  [task_time_s] -> Timer1/3
  [VDDM_LFSensorFailChk_flg] -> SR_Latch1/2(reset)
  SR_Latch1/1(latched) -> [VDDM_LFSensorFailPass_flg]
  Constant9/1 -> Equal6/2
  Equal6/1 -> SR_Latch1/1(set)
  Switch4/1 -> Logical Operator6/1, Timer1/2
  Switch6/1 -> Test Detection Criteria/1
  Constant12/1 -> Switch6/1
  [DTC_clear_request] -> Switch6/2
  Switch3/1 -> Switch6/3, [VDDM_LFSensorFailChk_flg]
  VTPM_LFSensorFail_flg/1 -> [VTPM_LFSensorFail_flg]
  Logical Operator4/1 -> Switch4/2
  Equal3/1 -> Logical Operator4/1
  [VPMM_PowerSta_enum] -> Equal2/1
  Constant3/1 -> Equal3/2
  Constant2/1 -> Equal2/2
  Constant8/1 -> Switch4/3
  Equal2/1 -> Logical Operator4/2
  [VPMM_PowerSta_enum] -> Equal3/1
  [task_time_s] -> Test Detection Criteria/2
  Constant/1 -> Test Detection Criteria/3
  Constant6/1 -> Test Detection Criteria/4
  [VPMM_PowerSta_enum] -> Equal5/1
  Equal1/1 -> Logical Operator1/2
  Equal5/1 -> Logical Operator1/1
  Logical Operator1/1 -> Switch3/2
  Constant7/1 -> Equal5/2
  Constant5/1 -> Equal1/2
  Constant4/1 -> Switch3/3
  [VPMM_PowerSta_enum] -> Equal1/1
  [DTC_clear_request] -> DTC_Info/4
  [VDDM_LFSensorFailPass_flg] -> DTC_Info/2
  [VDDM_LFSensorFailDet_flg] -> DTC_Info/1
  Test Detection Criteria/1 -> [VDDM_LFSensorFailDet_flg]  "VDDM_LFSensorFailDet_flg"
  DTC_Info/1 -> VDDM_LFSensorFailDTC_raw32/1  "VDDM_LFSensorFailDTC_raw32"
  [VDDM_LFSensorFailCFS_flg] -> DTC_Info/3
  [VPMM_PowerSta_enum] -> Equal4/1
  DTC_clear_request/1 -> [DTC_clear_request]
  [VDDM_LFSensorFailCFSRls_flg] -> Logical Operator3/3
  Logical Operator18/1 -> [VDDM_LFSensorFailCFS_flg]
  Constant14/1 -> Logical Operator12/1
  SR_Latch3/1 -> Logical Operator12/2
  Constant13/1 -> Logical Operator18/2
  Logical Operator12/1 -> [VDDM_LFSensorFailDFS_flg]
  SR_Latch4/1 -> Logical Operator18/1
  [VDDM_LFSensorFailCFSRls_flg] -> Logical Operator5/1
  [VDDM_LFSensorFailPass_flg] -> Logical Operator3/2
  DTC_Couter/1 -> SR_Latch4/1
  Data Type Conversion1/1 -> [VDDM_LFSensorFailDTC_cnt]  "VDDM_LFSensorFailDTC_cnt"
  Constant46/1 -> Logical Operator19/2
  Logical Operator19/1 -> DTC_Couter/1
  Constant11/1 -> Logical Operator15/2
  Logical Operator15/1 -> DTC_Couter/2
  Constant1/1 -> DTC_Couter/3
  DTC_Couter/2 -> Data Type Conversion1/1
  Relay/1 -> SR_Latch3/1
  [VDDM_LFSensorFailDet_flg] -> Logical Operator19/1
  Logical Operator3/1 -> Logical Operator15/1
  [VDDM_LFSensorFailCFS_flg] -> Logical Operator7/1
  [VDDM_LFSensorFailDTC_cnt] -> Relay/1
  Equal4/1 -> Logical Operator8/1
  Constant10/1 -> Equal4/2
  Constant24/1 -> Switch2/1
  [DTC_clear_request] -> Logical Operator8/2
  Switch2/1 -> [VDDM_LFSensorFailCFSRls_flg]
  Constant25/1 -> Switch2/3
  Logical Operator8/1 -> Switch2/2
  VPMM_PowerSta_enum/1 -> [VPMM_PowerSta_enum]
  task_time_s/1 -> [task_time_s]
  [VTPM_LFSensorFail_flg] -> Switch3/1
  [VTPM_LFSensorFail_flg] -> Switch4/1
  Logical Operator2/1 -> Logical Operator19/3
  [DTC_clear_request] -> Logical Operator3/1, Logical Operator2/1
  Logical Operator5/1 -> SR_Latch4/2
  [DTC_clear_request] -> Logical Operator5/2
  Logical Operator7/1 -> SR_Latch3/2
  [DTC_clear_request] -> Logical Operator7/2

== system ddm/DDM/DDM/TPM/LFWheelTmpHigh ==
  note: Test Detection Criteria
  note: Test Pass Criteria
  note: Release Condition After Decision
  note: Diagnostics and Fault Handling
  task_time_s : Inport
  VPMM_PowerSta_enum : Inport  Port=2
  DTC_clear_request : Inport  Port=3
  VTPM_LFWheelTmpHigh_flg : Inport  Port=4
  Constant : Constant  Value=KDDM_LFWheelTmpHighDTC_cnt
  Constant1 : Constant  Value=KDDM_LFWheelTmpHighDTC_cnt
  Constant10 : Constant  Value=ENUM_POWERSTA_OFF
  Constant11 : Constant  Value=KDDM_LFWheelTmpHighPassSW_flg
  Constant12 : Constant  Value=FALSE
  Constant13 : Constant  Value=KDDM_LFWheelTmpHighCFSSW_flg
  Constant14 : Constant  Value=KDDM_LFWheelTmpHighDFSSW_flg
  Constant15 : Constant  Value=KDDM_LFWheelTmpHighPassTO_s
  Constant2 : Constant  Value=ENUM_POWERSTA_READY
  Constant24 : Constant  Value=TRUE
  Constant25 : Constant  Value=FALSE
  Constant3 : Constant  Value=ENUM_POWERSTA_ON
  Constant4 : Constant  Value=FALSE
  Constant46 : Constant  Value=KDDM_LFWheelTmpHighDetSW_flg
  Constant5 : Constant  Value=ENUM_POWERSTA_READY
  Constant6 : Constant  Value=KDDM_LFWheelTmpHighDetTO_s
  Constant7 : Constant  Value=ENUM_POWERSTA_ON
  Constant8 : Constant  Value=TRUE
  Constant9 : Constant  Value=KDDM_LFWheelTmpHighPassTO_s
  DTC_Couter : hcu_lib/Basic_Blocks/DTC_Couter
  DTC_Info : hcu_lib/Basic_Blocks/DTC_Info
  Data Type Conversion1 : DataTypeConversion  OutDataTypeStr=uint8
  Equal{1..5} (5 alike) : RelationalOperator  Operator===  OutDataTypeStr=boolean  RndMeth=Simplest
  Equal6 : RelationalOperator  OutDataTypeStr=boolean  RndMeth=Simplest
  Logical Operator{1,4..5,7..8} (5 alike) : Logic  Operator=OR  AllPortsSameDT=off  OutDataTypeStr=boolean
  Logical Operator12 : Logic  AllPortsSameDT=off  OutDataTypeStr=boolean
  Logical Operator15 : Logic  AllPortsSameDT=off  OutDataTypeStr=boolean
  Logical Operator18 : Logic  AllPortsSameDT=off  OutDataTypeStr=boolean
  Logical Operator19 : Logic  Inputs=3  AllPortsSameDT=off  OutDataTypeStr=boolean
  Logical Operator2 : Logic  Operator=NOT  AllPortsSameDT=off  OutDataTypeStr=boolean
  Logical Operator3 : Logic  Operator=OR  Inputs=3  AllPortsSameDT=off  OutDataTypeStr=boolean
  Logical Operator6 : Logic  Operator=NOT  AllPortsSameDT=off  OutDataTypeStr=boolean
  Relay : Relay  OnSwitchValue=ONE_INT  OffSwitchValue=ZERO_INT
  SR_Latch1 : Subsystem  mask(SR_Latch){}
      mask help: SR latch function.
  SR_Latch3 : hcu_lib/Basic_Blocks/SR_Latch
  SR_Latch4 : hcu_lib/Basic_Blocks/SR_Latch
  Switch{2..4,6} (4 alike) : Switch  Criteria=u2 ~= 0
  Test Detection Criteria : hcu_lib/Basic_Blocks/Test Detection Criteria
  Timer1 : hcu_lib/Basic_Blocks/Timer
  VDDM_LFWheelTmpHighDTC_raw32 : Outport
  wires:
  [VTPM_LFWheelTmpHigh_flg] -> Switch4/1
  [VTPM_LFWheelTmpHigh_flg] -> Switch3/1
  task_time_s/1 -> [task_time_s]
  VPMM_PowerSta_enum/1 -> [VPMM_PowerSta_enum]
  Logical Operator8/1 -> Switch2/2
  Constant25/1 -> Switch2/3
  Switch2/1 -> [VDDM_LFWheelTmpHighCFSRls_flg]
  [DTC_clear_request] -> Logical Operator8/2
  Constant24/1 -> Switch2/1
  Constant10/1 -> Equal4/2
  Equal4/1 -> Logical Operator8/1
  [VDDM_LFWheelTmpHighDTC_cnt] -> Relay/1
  [VDDM_LFWheelTmpHighCFS_flg] -> Logical Operator7/1
  Logical Operator3/1 -> Logical Operator15/1
  [VDDM_LFWheelTmpHighDet_flg] -> Logical Operator19/1
  Relay/1 -> SR_Latch3/1
  DTC_Couter/2 -> Data Type Conversion1/1
  Constant1/1 -> DTC_Couter/3
  Logical Operator15/1 -> DTC_Couter/2
  Constant11/1 -> Logical Operator15/2
  Logical Operator19/1 -> DTC_Couter/1
  Constant46/1 -> Logical Operator19/2
  Data Type Conversion1/1 -> [VDDM_LFWheelTmpHighDTC_cnt]  "VDDM_LFWheelTmpHighDTC_cnt"
  DTC_Couter/1 -> SR_Latch4/1
  [VDDM_LFWheelTmpHighPass_flg] -> Logical Operator3/2
  [VDDM_LFWheelTmpHighCFSRls_flg] -> Logical Operator5/1
  SR_Latch4/1 -> Logical Operator18/1
  Logical Operator12/1 -> [VDDM_LFWheelTmpHighDFS_flg]
  Constant13/1 -> Logical Operator18/2
  SR_Latch3/1 -> Logical Operator12/2
  Constant14/1 -> Logical Operator12/1
  Logical Operator18/1 -> [VDDM_LFWheelTmpHighCFS_flg]
  [VDDM_LFWheelTmpHighCFSRls_flg] -> Logical Operator3/3
  DTC_clear_request/1 -> [DTC_clear_request]
  [VPMM_PowerSta_enum] -> Equal4/1
  [VDDM_LFWheelTmpHighCFS_flg] -> DTC_Info/3
  DTC_Info/1 -> VDDM_LFWheelTmpHighDTC_raw32/1  "VDDM_LFWheelTmpHighDTC_raw32"
  Test Detection Criteria/1 -> [VDDM_LFWheelTmpHighDet_flg]  "VDDM_LFWheelTmpHighDet_flg"
  [VDDM_LFWheelTmpHighDet_flg] -> DTC_Info/1
  [VDDM_LFWheelTmpHighPass_flg] -> DTC_Info/2
  [DTC_clear_request] -> DTC_Info/4
  [VPMM_PowerSta_enum] -> Equal1/1
  Constant4/1 -> Switch3/3
  Constant5/1 -> Equal1/2
  Constant7/1 -> Equal5/2
  Logical Operator1/1 -> Switch3/2
  Equal5/1 -> Logical Operator1/1
  Equal1/1 -> Logical Operator1/2
  [VPMM_PowerSta_enum] -> Equal5/1
  Constant6/1 -> Test Detection Criteria/4
  Constant/1 -> Test Detection Criteria/3
  [task_time_s] -> Test Detection Criteria/2
  [VPMM_PowerSta_enum] -> Equal3/1
  Equal2/1 -> Logical Operator4/2
  Constant8/1 -> Switch4/3
  Constant2/1 -> Equal2/2
  Constant3/1 -> Equal3/2
  [VPMM_PowerSta_enum] -> Equal2/1
  Equal3/1 -> Logical Operator4/1
  Logical Operator4/1 -> Switch4/2
  VTPM_LFWheelTmpHigh_flg/1 -> [VTPM_LFWheelTmpHigh_flg]
  Switch3/1 -> [VDDM_LFWheelTmpHighChk_flg], Switch6/3
  [DTC_clear_request] -> Switch6/2
  Constant12/1 -> Switch6/1
  Switch6/1 -> Test Detection Criteria/1
  Switch4/1 -> Timer1/2, Logical Operator6/1
  Equal6/1 -> SR_Latch1/1(set)
  Constant9/1 -> Equal6/2
  SR_Latch1/1(latched) -> [VDDM_LFWheelTmpHighPass_flg]
  [VDDM_LFWheelTmpHighChk_flg] -> SR_Latch1/2(reset)
  [task_time_s] -> Timer1/3
  Timer1/1 -> Equal6/1
  Constant15/1 -> Timer1/4
  Logical Operator6/1 -> Timer1/1
  Logical Operator2/1 -> Logical Operator19/3
  [DTC_clear_request] -> Logical Operator3/1, Logical Operator2/1
  Logical Operator5/1 -> SR_Latch4/2
  [DTC_clear_request] -> Logical Operator5/2
  Logical Operator7/1 -> SR_Latch3/2
  [DTC_clear_request] -> Logical Operator7/2
